simulink model "RF_FrontEnd_final"  (R2012b)
settings: Solver=FixedStepDiscrete  SolverMode=SingleTasking  StartTime=0.0  StopTime=4e-4  RelTol=1e-3
model workspace (MAT data in the model file):
  Ts = 1.6667e-07
  mf_lfm = [-0.999229036241+0.0392598157591i; 0.987688340595-0.15643446504i; -0.938191335922+0.346117057077i; 0.809016994375-0.587785252292i; -0.55557023302+0.831469612303i; 0.15643446504-0.987688340595i; 0.346117057077+0.938191335922i; -0.809016994375-0.587785252292i; 0.999229036241-0.0392598157591i; -0.707106781187+0.707106781187i; -0.0392598157591-0.999229036241i; 0.809016994375+0.587785252292i; -0.938191335922+0.346117057077i; 0.15643446504-0.987688340595i; 0.831469612303+0.55557023302i; -0.809016994375+0.587785252292i; -0.346117057077-0.938191335922i; 0.987688340595-0.15643446504i; 0.0392598157591+0.999229036241i; -1-6.12323399574e-16i; -0.0392598157591-0.999229036241i; 0.987688340595-0.15643446504i; 0.346117057077+0.938191335922i; -0.809016994375+0.587785252292i; -0.831469612303-0.55557023302i; 0.15643446504-0.987688340595i; 0.938191335922-0.346117057077i; 0.809016994375+0.587785252292i; 0.0392598157591+0.999229036241i; -0.707106781187+0.707106781187i; -0.999229036241+0.0392598157591i; -0.809016994375-0.587785252292i; -0.346117057077-0.938191335922i; 0.15643446504-0.987688340595i; 0.55557023302-0.831469612303i; 0.809016994375-0.587785252292i; 0.938191335922-0.346117057077i; 0.987688340595-0.15643446504i; 0.999229036241-0.0392598157591i; 1+0i]
  carrierFreq = 2100000000
values from neighbouring files (symbols this model uses):
  Cs = [1.14512e-11 3.76384e-13 1.14512e-11]    [RF_FrontEnd.mat]
  iFreq = 70000000    [RF_FrontEnd.mat]
  Ls = [4.62272e-10 1.406368e-08 4.62272e-10]    [RF_FrontEnd.mat]
undefined symbols (not defined in the file or in its folder): dBc, dfilt, Hz, magnitude, read, rfdata
libraries: dspstat3 x4, rfports1 x2, rfamplifiers1 x2, dspmathops x2, rfladderfilters1 x1, rfmixers1 x1, dsparch4 x1, dspsrcs4 x1
settings Model: Creator=jbryan  LastModifiedBy=jbryan
settings DataIOCC: SignalLoggingSaveFormat=ModelDataLogs  SaveOutput=off  SignalLogging=off  SaveTime=off
settings DebuggingCC: AlgebraicLoopMsg=error  SingleTaskRateTransMsg=error  FcnCallInpInsideContextMsg=UseLocalSettings  StrictBusMsg=Warning
settings GRTTargetCC: CombineOutputUpdateFcns=off  GRTInterface=on

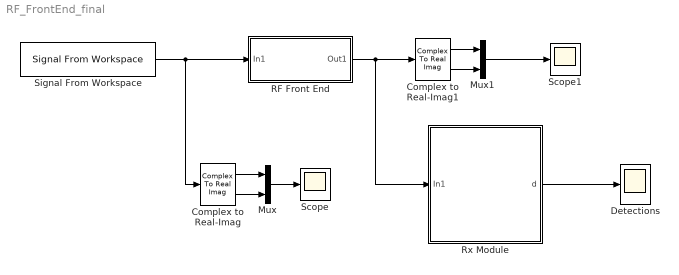
== system RF_FrontEnd_final ==
  Complex to Real-Imag : ComplexToRealImag
  Complex to Real-Imag1 : ComplexToRealImag
  Detections : Scope
      settings: TimeRange=0.005  YMin=0  YMax=1  SaveName=ScopeData2
  Mux : Mux  Inputs=2
  Mux1 : Mux  Inputs=2
  RF Front End : Subsystem
  Rx Module : Subsystem
      mask Display: image(imread('RxBoard1.jpg'))
  Scope : Scope
  Scope1 : Scope
      settings: YMin=-0.0004  YMax=0.00035
  Signal From Workspace : dspsrcs4/Signal From Workspace  X=targetReturn  Ts=Ts  nsamps=1  OutputAfterFinalValue=Cyclic repetition  ignoreOrWarnInputAndFrameLengths=off
  wires:
  Complex to Real-Imag/1 -> Mux/1
  Complex to Real-Imag/2 -> Mux/2
  Mux/1 -> Scope/1
  Signal From Workspace/1 -> Complex to Real-Imag/1, RF Front End/1(In1)
  Complex to Real-Imag1/1 -> Mux1/1
  Complex to Real-Imag1/2 -> Mux1/2
  Mux1/1 -> Scope1/1
  RF Front End/1(Out1) -> Rx Module/1(In1), Complex to Real-Imag1/1
  Rx Module/1(d) -> Detections/1

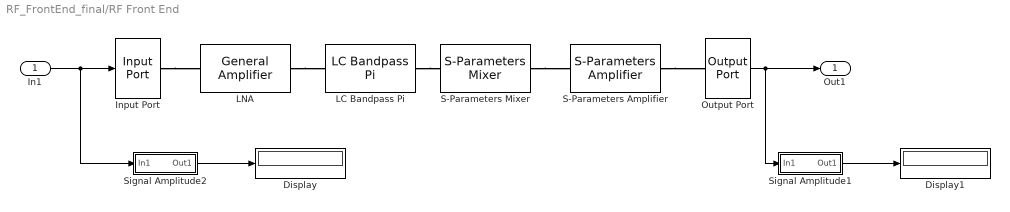
== system RF_FrontEnd_final/RF Front End ==
  In1 : Inport
  Display : Display
  Display1 : Display
  Input Port : rfports1/Input Port  Description=source block  TreatSimulinkInputSignalAs=Incident power wave  MaxLength=128  FracBW=0  ModelDelay=0  Fc=carrierFreq  Ts=Ts  Zs=50  RFhasDSP=Columns as channels (frame based)  NoiseFlag=on  seed=67987  GoToTag=ABDCCBARCBJSOUIPGBSKSHY
  LC Bandpass Pi : rfladderfilters1/LC Bandpass Pi  LConnTagsString=__newl0  RConnTagsString=__newr0  L=Ls  C=Cs  PlotFreq=User-specified  SourceFreq=User-specified  Freq=[0:100e6:3e9]  AllPlotType=X-Y plane  AppliedNetworkData=S21  AppliedComplexFormat=Magnitude (decibels)  AppliedNetworkData2=""  AppliedXParameter=Freq  AppliedXFormat=Hz  YOption=Linear  XOption=Linear  PlotZ0=50  DisplayData=off  PlotFreqNoSim=User-specified  NetworkData=S21  SmithData=S11  PolarData=S11  ComplexFormat=Magnitude (decibels)  DBFormat=Magnitude (decibels)  NoneFormat=None
  LNA : rfamplifiers1/General Amplifier  LConnTagsString=__newl0  RConnTagsString=__newr0  DataSource=Data file  RFDATA=read(rfdata.data, 'default.amp')  File=max2641.s2p  InterpMethod=Linear  IP3Type=OIP3  IIP3=inf  OIP3=inf  P1dB=inf  PSat=inf  GCSat=0  NonlinearDataFreq=2.0e9  NoiseDefinedBy=Noise figure  NF=0  FMIN=0  GammaOpt=1+0i  RN=1  NFactor=1  NTemp=0  NoiseDataFreq=2.0e9  PlotFreq=Extracted from RFDATA object  SourceFreq=Extracted from data source  Freq=[1e9:1e8:2.9e9]  SourcePin=Extracted from data source  Pin=[0:19]  AllPlotType=X-Y plane  AppliedNetworkData=S11  AppliedComplexFormat=Magnitude (decibels)  AppliedNetworkData2=""  AppliedComplexFormat2=""  AppliedXParameter=Freq  AppliedXFormat=Auto  YOption=Linear  XOption=Linear  ConditionNames=Bias!  ConditionValues=1.9!  PlotZ0=50  PlotFreqNoSim=User-specified  DisplayData=off  NetworkData=S11  SmithData=S11  PolarData=S11  ComplexFormat=Magnitude (decibels)  DBFormat=Magnitude (decibels)  NoneFormat=None  PowerData=0  PowerFormat=0  PhaseFormat=0
  Output Port : rfports1/Output Port  Zl=50  Flag=0  num_Models=0  GoToTag=ABDCCBARCBJSOUIPGBSKSHY  PlotFreq=User-specified  SourceFreq=Derived from Input Port parameters  Freq=1e9:1e8:3e9  AllPlotType=X-Y plane  AppliedNetworkData=S21  AppliedComplexFormat=Magnitude (decibels)  AppliedNetworkData2=NF  AppliedComplexFormat2=Magnitude (decibels)  AppliedXParameter=Freq  AppliedXFormat=Hz  YOption=Linear  XOption=Linear  PlotZ0=50  DisplayData=off  NoBudgetPlot=Composite data  NetworkData=S11  SmithData=S11  PolarData=S11  ComplexFormat=Magnitude (decibels)  DBFormat=Magnitude (decibels)  DBMFormat=dBm  NoneFormat=None
  S-Parameters Amplifier : rfamplifiers1/S-Parameters Amplifier  LConnTagsString=__newl0  RConnTagsString=__newr0  NetParamData=[0,0;sqrt(1000),0]  NetParamFreq=iFreq  Z0=50  InterpMethod=Linear  IP3Type=OIP3  IIP3=inf  OIP3=100  P1dB=inf  PSat=inf  GCSat=0  NonlinearDataFreq=2.0e9  NoiseDefinedBy=Noise figure  NF=20  FMIN=0  GammaOpt=1  RN=1  NFactor=1  NTemp=0  NoiseDataFreq=2.0e9  PlotFreq=Derived from Input Port parameters  SourceFreq=Same as the s-parameters frequency  Freq=[1.9e9:1.0e8:2.2e9]  SourcePin=Extracted from data source  Pin=0  AllPlotType=X-Y plane  AppliedNetworkData=S11  AppliedComplexFormat=Magnitude (decibels)  AppliedNetworkData2=""  AppliedXParameter=Freq  AppliedXFormat=Hz  YOption=Linear  XOption=Linear  PlotZ0=50  PlotFreqNoSim=User-specified  DisplayData=off  NetworkData=S11  SmithData=S11  PolarData=S11  ComplexFormat=Magnitude (decibels)  DBFormat=Magnitude (decibels)  NoneFormat=None
  S-Parameters Mixer : rfmixers1/S-Parameters Mixer  LConnTagsString=__newl0  RConnTagsString=__newr0  NetParamData=[0,0;1,0]  NetParamFreq=2.0e9  Z0=50  InterpMethod=Linear  MixerType=Downconverter  FLO=carrierFreq-iFreq  IP3Type=OIP3  IIP3=inf  OIP3=100  P1dB=inf  PSat=inf  GCSat=0  NonlinearDataFreq=2.0e9  NoiseDefinedBy=Noise figure  NF=10  FMIN=0  GammaOpt=1  RN=1  NFactor=1  NTemp=0  NoiseDataFreq=2.0e9  FreqOffset=[0.1 1 10 100]*1e3  PhaseNoiseLevel=[-70 -120 -140 -150]  PlotFreq=Same as the Frequency parameter  SourceFreq=Same as the s-parameters frequency  Freq=[1e9:1e8:2.9e9]  SourcePin=Extracted from data source  Pin=0  AllPlotType=X-Y plane  AppliedNetworkData=S11  AppliedComplexFormat=Magnitude (decibels)  AppliedNetworkData2=""  AppliedXParameter=Freq  AppliedXFormat=Hz  YOption=Linear  XOption=Linear  PlotZ0=50  PlotFreqNoSim=User-specified  DisplayData=off  NetworkData=S11  SmithData=S11  PolarData=S11  ComplexFormat=Magnitude (decibels)  DBFormat=Magnitude (decibels)  NoneFormat=None  DBcFormat=dBc/Hz
  Signal Amplitude1 : Subsystem
  Signal Amplitude2 : Subsystem
  Out1 : Outport
  wires:
  In1/1 -> Input Port/1, Signal Amplitude2/1(In1)
  Output Port/1 -> Out1/1, Signal Amplitude1/1(In1)
  Signal Amplitude2/1(Out1) -> Display/1
  Signal Amplitude1/1(Out1) -> Display1/1
  connections:
  Input Port/RConn1 -- LNA/LConn1
  S-Parameters Amplifier/RConn1 -- Output Port/LConn1
  LNA/RConn1 -- LC Bandpass Pi/LConn1
  LC Bandpass Pi/RConn1 -- S-Parameters Mixer/LConn1
  S-Parameters Mixer/RConn1 -- S-Parameters Amplifier/LConn1

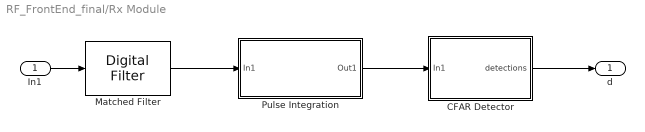
== system RF_FrontEnd_final/Rx Module ==
  In1 : Inport
  CFAR Detector : Subsystem  mask(Cell Averaging CFAR){WindowLength=31, GuardLength=5, Pfa=1e-6}
      mask prompts: WindowLength "Window Length"; GuardLength "Guard cells (per side)"; Pfa "Probability of false alarm"
      mask help: Cell averaging CFAR. Specify the window length, the number of guard cells on each side of the cell under test, and the probability of false alarm.
      mask init:
      | N = WindowLength - 2*GuardLength - 1;
  Matched Filter : dsparch4/Digital Filter  TypePopup=FIR (all zeros)  IIRFiltStruct=Direct form II transposed  AllPoleFiltStruct=Direct form  FIRFiltStruct=Direct form  CoeffSource=Specify via dialog  NumCoeffs=mf_lfm  DenCoeffs=[1 0.1]  BiQuadCoeffs=[1 0.3 0.4 1 0.1 0.2]  LatticeCoeffs=[0.2 0.4]  denIgnore=on  FiltPerSampPopup=One filter per frame  IC=0  ICnum=0  ICden=0  roundingMode=Floor  overflowMode=off  ScaleValues=1  scaleValueFracLength=14  stageInFracLength=15  stageOutFracLength=15  FilterSource=Specify via dialog  dfiltObjectName=dfilt.dffir([1 2 1])  InputProcessing=Columns as channels (frame based)
  Pulse Integration : Subsystem  mask(Noncoherent pulse integration){pulseLen=200, N=10}
      mask prompts: pulseLen "Pulse length (samples)"; N "Number of pulses"
  d : Outport
  wires:
  In1/1 -> Matched Filter/1
  Matched Filter/1 -> Pulse Integration/1(In1)
  Pulse Integration/1(Out1) -> CFAR Detector/1(In1)
  CFAR Detector/1(detections) -> d/1

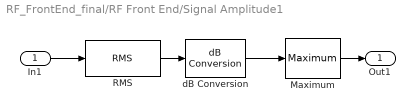
== system RF_FrontEnd_final/RF Front End/Signal Amplitude1 ==
  In1 : Inport
  Maximum : dspstat3/Maximum  fcn=Running  reset=None  InputProcessing=Inherited (this choice will be removed - see release notes)  indexBase=One  operateOver=Each column  Dimension=1  colComp=on  operation=maximum  roiEnable=off  roiType=Rectangles  roiPortion=Entire ROI  roiOutput=Individual statistics for each ROI  roiFlag=off  accumDataTypeStr=Inherit: Same as product output  accumLastDataTypeStr=Inherit: Same as product output  roundingMode=Floor  overflowMode=off
  RMS : dspstat3/RMS  run=off  reset_popup=None  InputProcessing=Columns as channels (frame based)  directionMode=Each column  dimension=1  treatSBRowAsCol=on
  dB Conversion : dspmathops/dB Conversion  dBtype=dB  intype=Amplitude  R=1  fuzz=off
  Out1 : Outport
  wires:
  dB Conversion/1 -> Maximum/1
  RMS/1 -> dB Conversion/1
  In1/1 -> RMS/1
  Maximum/1 -> Out1/1

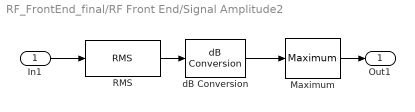
== system RF_FrontEnd_final/RF Front End/Signal Amplitude2 ==
  In1 : Inport
  Maximum : dspstat3/Maximum  fcn=Running  reset=None  InputProcessing=Inherited (this choice will be removed - see release notes)  indexBase=One  operateOver=Each column  Dimension=1  colComp=on  operation=maximum  roiEnable=off  roiType=Rectangles  roiPortion=Entire ROI  roiOutput=Individual statistics for each ROI  roiFlag=off  accumDataTypeStr=Inherit: Same as product output  accumLastDataTypeStr=Inherit: Same as product output  roundingMode=Floor  overflowMode=off
  RMS : dspstat3/RMS  run=off  reset_popup=None  InputProcessing=Columns as channels (frame based)  directionMode=Each column  dimension=1  treatSBRowAsCol=on
  dB Conversion : dspmathops/dB Conversion  dBtype=dB  intype=Amplitude  R=1  fuzz=off
  Out1 : Outport
  wires:
  Maximum/1 -> Out1/1
  In1/1 -> RMS/1
  RMS/1 -> dB Conversion/1
  dB Conversion/1 -> Maximum/1

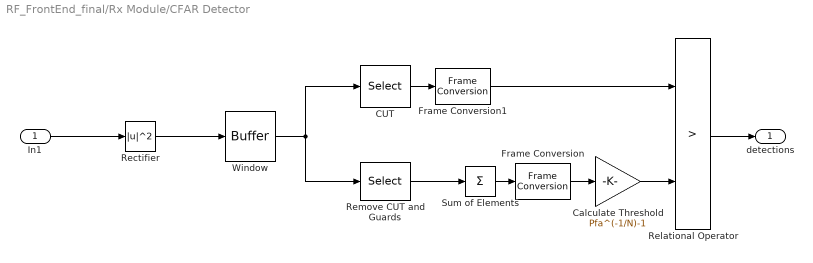
== system RF_FrontEnd_final/Rx Module/CFAR Detector ==
  In1 : Inport
  CUT : Selector  InputPortWidth=WindowLength  IndexOptions=Index vector (dialog)  Indices=ceil(WindowLength/2)  OutputSizes=1
  Calculate Threshold : Gain  Gain=Pfa^(-1/N)-1
  Frame Conversion : FrameConversion  OutFrame=Sample-based
  Frame Conversion1 : FrameConversion  OutFrame=Sample-based
  Rectifier : Math  Operator=magnitude^2  SaturateOnIntegerOverflow=on
  Relational Operator : RelationalOperator  Operator=>  OutDataTypeStr=float('double')
  Remove CUT and Guards : Selector  InputPortWidth=WindowLength  IndexOptions=Index vector (dialog)  Indices=[1:N/2,(WindowLength-N/2+1):WindowLength]  OutputSizes=1
  Sum of Elements : Sum  Inputs=+
  Window : Buffer  N=WindowLength  V=WindowLength-1  TreatMby1Signals=One channel
  detections : Outport
  wires:
  In1/1 -> Rectifier/1
  Window/1 -> CUT/1, Remove CUT and Guards/1
  Rectifier/1 -> Window/1
  Remove CUT and Guards/1 -> Sum of Elements/1
  Sum of Elements/1 -> Frame Conversion/1
  Frame Conversion/1 -> Calculate Threshold/1
  CUT/1 -> Frame Conversion1/1
  Calculate Threshold/1 -> Relational Operator/2
  Frame Conversion1/1 -> Relational Operator/1
  Relational Operator/1 -> detections/1

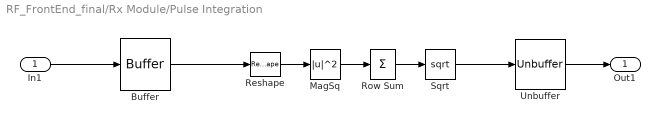
== system RF_FrontEnd_final/Rx Module/Pulse Integration ==
  In1 : Inport
  Buffer : Buffer  N=pulseLen*N  V=pulseLen*(N-1)  TreatMby1Signals=One channel
  MagSq : Math  Operator=magnitude^2  SaturateOnIntegerOverflow=on
  Reshape : Reshape  OutputDimensionality=Customize  OutputDimensions=[200,10]
  Row Sum : Sum  Inputs=+  CollapseMode=Specified dimension  CollapseDim=2
  Sqrt : Sqrt  SaturateOnIntegerOverflow=on
  Unbuffer : Unbuffer  SampleBasedProcessing=Same as frame based
  Out1 : Outport
  wires:
  MagSq/1 -> Row Sum/1
  Reshape/1 -> MagSq/1
  In1/1 -> Buffer/1
  Row Sum/1 -> Sqrt/1
  Buffer/1 -> Reshape/1
  Unbuffer/1 -> Out1/1
  Sqrt/1 -> Unbuffer/1
